simulink model "rlc_gformer"  (R2017b)
settings: Solver=VariableStepAuto  StartTime=0.0  StopTime=0.08  MaxStep=1e-4  RelTol=1e-3
values from neighbouring files (symbols this model uses):
  C_m = 1e-6    (= 1e-06)    [rlc_gformer_ini.m]
  F_b = 50.0    (= 50)    [rl2_ini.m]    (also in rl_ini.m; rl_ini_jm.m; rlc_gformer_ini.m)
  L_l = 1e-3    (= 0.001)    [rlc_gformer_ini.m]
  L_t = 5e-3    (= 0.005)    [rlc_gformer_ini.m]
  R_l = 1.0    (= 1)    [rlc_gformer_ini.m]
  R_m = 26.0    (= 26)    [rlc_gformer_ini.m]
  R_t = 1.0    (= 1)    [rlc_gformer_ini.m]
undefined symbols (not defined in the file or in its folder): C_, DiscIntNeverNeededParam, K_i, K_p, L_s, R_s, T_s_power, vsc_ini
libraries: powerlib x11, powerlib_meascontrol x8
settings Model: Creator=jmmauricio  LastModifiedBy=jmmau
settings CodeAppCC: StateflowObjectComments=on
settings SimscapeCC: SimscapeNormalizeSystem=off

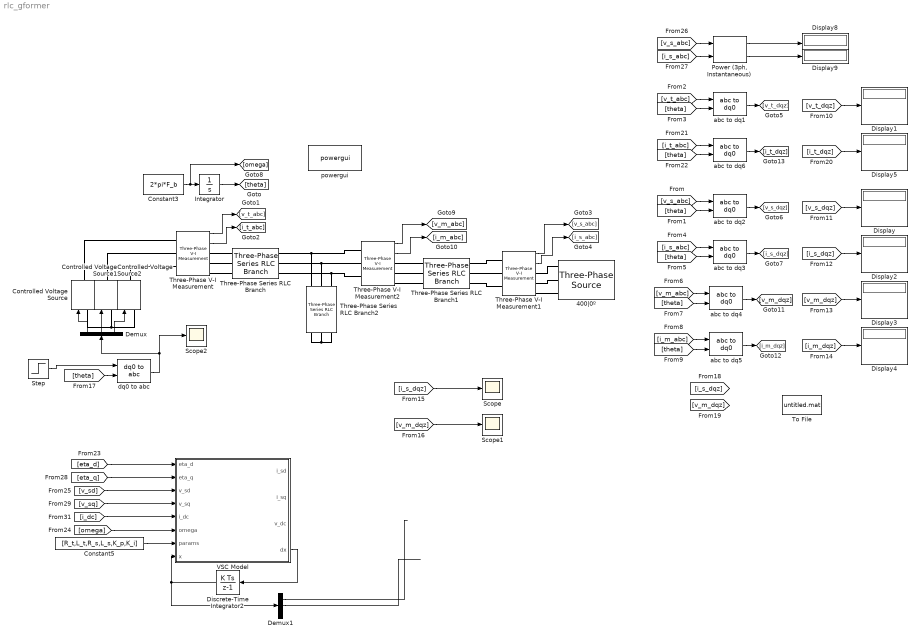
== system rlc_gformer ==
  400|0º : powerlib/Electrical Sources/Three-Phase Source  InternalConnection=Yg  VoltagePhases=off  Voltage=400  PhaseAngle=0  Voltage_phases=[25e3 25e3 25e3]/sqrt(3)  PhaseAngles_phases=[0 -120 +120]  Frequency=50  NonIdealSource=off  SpecifyImpedance=off  Resistance=0.8929  Inductance=16.58e-3  ShortCircuitLevel=100e6  BaseVoltage=25e3  XRratio=7  BusType=swing  Pref=10e3  Qref=0  Prefabc=[10e3, 10e3, 10e3]  Qrefabc=[0, 0, 0]  Qmin=-inf  Qmax=inf
  Constant3 : Constant  Value=2*pi*F_b
  Constant5 : Constant  Value=[R_t,L_t,R_s,L_s,K_p,K_i]
  Controlled Voltage Source : powerlib/Electrical Sources/Controlled Voltage Source  Initialize=on  Source_Type=AC  Amplitude=0  Phase=0  Frequency=0  Measurements=None
  Controlled Voltage Source1 : powerlib/Electrical Sources/Controlled Voltage Source  Initialize=on  Source_Type=AC  Amplitude=0  Phase=0  Frequency=0  Measurements=None
  Controlled Voltage Source2 : powerlib/Electrical Sources/Controlled Voltage Source  Initialize=on  Source_Type=AC  Amplitude=0  Phase=0  Frequency=0  Measurements=None
  Demux : Demux  Outputs=3
  Demux1 : Demux  Outputs=3
  Discrete-Time Integrator2 : DiscreteIntegrator  InitialCondition=vsc_ini  InitialConditionSetting=State (most efficient)  SampleTime=T_s_power  ICPrevOutput=DiscIntNeverNeededParam  ICPrevScaledInput=DiscIntNeverNeededParam
  Display{,1..5,8..9} (8 alike) : Display
  Integrator : Integrator
  "Power (3ph, Instantaneous)" : powerlib_meascontrol/Measurements/Power (3ph, Instantaneous)
      settings: SourceProductName=Simscape Power Systems
  Scope : Scope
  Scope1 : Scope
  Scope2 : Scope
  Step : Step  Time=0.02  Before=[0,-400*sqrt(2/3),0]  After=[100,-400*sqrt(2/3)*1.1,0]  SampleTime=0
  Three-Phase Series RLC Branch : powerlib/Elements/Three-Phase Series RLC Branch  LConnTagsString=A|B|C  RConnTagsString=A|B|C  BranchType=RL  Resistance=R_t  Inductance=L_t  Capacitance=1e-6  Measurements=None
  Three-Phase Series RLC Branch1 : powerlib/Elements/Three-Phase Series RLC Branch  LConnTagsString=A|B|C  RConnTagsString=A|B|C  BranchType=RL  Resistance=R_l  Inductance=L_l  Capacitance=1e-6  Measurements=None
  Three-Phase Series RLC Branch2 : powerlib/Elements/Three-Phase Series RLC Branch  LConnTagsString=A|B|C  RConnTagsString=A|B|C  BranchType=RC  Resistance=R_m  Inductance=C_  Capacitance=C_m  Measurements=None
  Three-Phase V-I Measurement : powerlib/Measurements/Three-Phase V-I Measurement  VoltageMeasurement=phase-to-ground  SetLabelV=off  LabelV=Vabc  Vpu=off  VpuLL=off  CurrentMeasurement=yes  SetLabelI=off  LabelI=Iabc  Ipu=off  Pbase=100e6  Vbase=500e3  OutputType=Complex  PhasorSimulation=off  PSBequivalent=0
  Three-Phase V-I Measurement1 : powerlib/Measurements/Three-Phase V-I Measurement  VoltageMeasurement=phase-to-ground  SetLabelV=off  LabelV=Vabc  Vpu=off  VpuLL=off  CurrentMeasurement=yes  SetLabelI=off  LabelI=Iabc  Ipu=off  Pbase=100e6  Vbase=500e3  OutputType=Complex  PhasorSimulation=off  PSBequivalent=0
  Three-Phase V-I Measurement2 : powerlib/Measurements/Three-Phase V-I Measurement  VoltageMeasurement=phase-to-ground  SetLabelV=off  LabelV=Vabc  Vpu=off  VpuLL=off  CurrentMeasurement=yes  SetLabelI=off  LabelI=Iabc  Ipu=off  Pbase=100e6  Vbase=500e3  OutputType=Complex  PhasorSimulation=off  PSBequivalent=0
  To File : ToFile  SaveFormat=Timeseries
  VSC Model : MATLAB Function  TreatAsAtomicUnit=on
  abc to dq{1..6} (6 alike) : powerlib_meascontrol/Transformations/abc to dq0  Alignment=Aligned with phase A axis
  dq0 to abc : powerlib_meascontrol/Transformations/dq0 to abc  Alignment=Aligned with phase A axis
  powergui : powerlib/powergui  Priority=1  SimulationMode=Continuous  SampleTime=T_s_power  frequency=60  Iterations=50  frequencyindice=50  Pbase=100e6  ErrMax=1e-4  UnitsV=kV  UnitsW=MW  buscounter=0  FunctionMessages=off  echomessages=off  EnableUseOfTLC=off  CurrentSourceSwitches=off  DisableSnubberDevices=off  DisableRonSwitches=off  DisableVfSwitches=off  DisplayEquations=off  SolverType=Tustin/Backward Euler (TBE)  Interpol=off  ExternalGateDelay=off  methode=off  Ts=100  x0status=zero  SPID=on  SwTol=0  HookPort=off  RestoreLinks=warning  ResistiveCurrentMeasurement=off  Frange=[0:2:500]  Ylog=off  Xlog=on  ShowGrid=off  save=off  variable=ZData  structure=0  ZoomFFT=off  StartTime=0.0  cycles=1  DisplayStyle=1  fundamental=60  FreqAxis=off  MaxFrequency=1000  frequencyindicesteady=1  RmsSteady=1  display=off
  wires:
  Constant3/1 -> [omega], Integrator/1
  Integrator/1 -> [theta]
  Three-Phase V-I Measurement/1 -> [v_t_abc]
  Three-Phase V-I Measurement/2 -> [i_t_abc]
  Three-Phase V-I Measurement1/2 -> [i_s_abc]
  Three-Phase V-I Measurement1/1 -> [v_s_abc]
  [v_s_abc] -> abc to dq2/1
  [theta] -> abc to dq2/2
  [v_t_abc] -> abc to dq1/1
  [theta] -> abc to dq1/2
  [i_s_abc] -> abc to dq3/1
  [theta] -> abc to dq3/2
  abc to dq1/1 -> [v_t_dqz]
  abc to dq2/1 -> [v_s_dqz]
  abc to dq3/1 -> [i_s_dqz]
  [v_t_dqz] -> Display1/1
  [v_s_dqz] -> Display/1
  [i_s_dqz] -> Display2/1
  [v_s_abc] -> "Power (3ph, Instantaneous)"/1
  [i_s_abc] -> "Power (3ph, Instantaneous)"/2
  "Power (3ph, Instantaneous)"/2 -> Display9/1
  "Power (3ph, Instantaneous)"/1 -> Display8/1
  Three-Phase V-I Measurement2/2 -> [i_m_abc]
  Three-Phase V-I Measurement2/1 -> [v_m_abc]
  abc to dq4/1 -> [v_m_dqz]
  abc to dq5/1 -> [i_m_dqz]
  [theta] -> abc to dq5/2
  [v_m_abc] -> abc to dq4/1
  [i_m_abc] -> abc to dq5/1
  [theta] -> abc to dq4/2
  [v_m_dqz] -> Display3/1
  [i_m_dqz] -> Display4/1
  [i_s_dqz] -> Scope/1
  [v_m_dqz] -> Scope1/1
  Demux/3 -> Controlled Voltage Source2/1
  Demux/2 -> Controlled Voltage Source1/1
  Demux/1 -> Controlled Voltage Source/1
  dq0 to abc/1 -> Scope2/1, Demux/1
  [theta] -> dq0 to abc/2
  Step/1 -> dq0 to abc/1
  abc to dq6/1 -> [i_t_dqz]
  [i_t_abc] -> abc to dq6/1
  [theta] -> abc to dq6/2
  [i_t_dqz] -> Display5/1
  Demux1/2 -> ?
  Constant5/1 -> VSC Model/7(params)
  [i_dc] -> VSC Model/5(i_dc)
  [eta_q] -> VSC Model/2(eta_q)
  [v_sq] -> VSC Model/4(v_sq)
  [eta_d] -> VSC Model/1(eta_d)
  [v_sd] -> VSC Model/3(v_sd)
  Demux1/1 -> ?
  VSC Model/4(dx) -> Discrete-Time Integrator2/1
  Discrete-Time Integrator2/1 -> VSC Model/8(x), Demux1/1
  [omega] -> VSC Model/6(omega)
  connections:
  Controlled Voltage Source/RConn1 -- Three-Phase V-I Measurement/LConn1
  Controlled Voltage Source1/RConn1 -- Three-Phase V-I Measurement/LConn2
  Controlled Voltage Source2/RConn1 -- Three-Phase V-I Measurement/LConn3
  Three-Phase Series RLC Branch/LConn1 -- Three-Phase V-I Measurement/RConn1
  Three-Phase Series RLC Branch/LConn2 -- Three-Phase V-I Measurement/RConn2
  Three-Phase Series RLC Branch/LConn3 -- Three-Phase V-I Measurement/RConn3
  Three-Phase V-I Measurement1/RConn3 -- 400|0º/RConn3
  Three-Phase V-I Measurement1/RConn2 -- 400|0º/RConn2
  Three-Phase V-I Measurement1/RConn1 -- 400|0º/RConn1
  Three-Phase Series RLC Branch/RConn1 -- Three-Phase Series RLC Branch2/LConn1 -- Three-Phase V-I Measurement2/LConn1
  Three-Phase Series RLC Branch/RConn2 -- Three-Phase Series RLC Branch2/LConn2 -- Three-Phase V-I Measurement2/LConn2
  Three-Phase Series RLC Branch/RConn3 -- Three-Phase Series RLC Branch2/LConn3 -- Three-Phase V-I Measurement2/LConn3
  Controlled Voltage Source/LConn1 -- Controlled Voltage Source1/LConn1 -- Controlled Voltage Source2/LConn1
  Three-Phase Series RLC Branch1/LConn2 -- Three-Phase V-I Measurement2/RConn2
  Three-Phase Series RLC Branch1/LConn3 -- Three-Phase V-I Measurement2/RConn3
  Three-Phase Series RLC Branch1/LConn1 -- Three-Phase V-I Measurement2/RConn1
  Three-Phase Series RLC Branch1/RConn1 -- Three-Phase V-I Measurement1/LConn1
  Three-Phase Series RLC Branch1/RConn2 -- Three-Phase V-I Measurement1/LConn2
  Three-Phase Series RLC Branch1/RConn3 -- Three-Phase V-I Measurement1/LConn3
  Three-Phase Series RLC Branch2/RConn1 -- Three-Phase Series RLC Branch2/RConn2 -- Three-Phase Series RLC Branch2/RConn3

== matlab function rlc_gformer/VSC Model ==
  data: eta_d input; eta_q input; i_sd output; i_sq output; v_dc output; v_sd input; v_sq input; i_dc input; omega input; params input; dx output; x input
function [i_sd,i_sq,v_dc,dx] = vsc_lc_dq(eta_d,eta_q,v_sd,v_sq,i_dc,omega,params,x)

% parameters
R_s  = params(1);
L_s  = params(2);
C_dc = params(3);

% from the integrator to the states
i_sd  = x(1);
i_sq  = x(2);
v_dc =  x(3);

% derivatives
di_sd  = 1/L_s*(v_td + L_s*omega*i_tq - R_s*i_sd - v_sd);
di_sq  = 1/L_s*(v_tq - L_s*omega*i_td - R_s*i_sq - v_sq);
di_sd  = 1/L_s*(v_md + L_s*omega*i_sq - R_s*i_sd - v_sd);
di_sq  = 1/L_s*(v_mq - L_s*omega*i_sd - R_s*i_sq - v_sq);
di_sd  = 1/L_s*(v_md + L_s*omega*i_sq - R_s*i_sd - v_sd);
di_sq  = 1/L_s*(v_mq - L_s*omega*i_sd - R_s*i_sq - v_sq);



% from derivatives to the integrator
dx = [di_sd,di_sq,dv_dc];
